simulink model "Template_v5_0_0_2024b_Jetson"  (R2024b)
settings: Solver=ode4  StartTime=0.0  StopTime=tsim  FixedStep=baseRate  RelTol=1e-6  AbsTol=1e-6
values from neighbouring files (symbols this model uses):
  Gamma1_el = 0.12    [Run_Initializer.m]
  Gamma1_sh = 0.005    [Run_Initializer.m]
  Gamma1_wr = 0.025    [Run_Initializer.m]
  Gamma2_el = 5    [Run_Initializer.m]
  Gamma2_sh = 5    [Run_Initializer.m]
  Gamma2_wr = 5    [Run_Initializer.m]
  Gamma3_el = 10    [Run_Initializer.m]
  Gamma3_sh = 40    [Run_Initializer.m]
  Gamma3_wr = 40    [Run_Initializer.m]
  Gamma4_el = 0.039    [Run_Initializer.m]
  Gamma4_sh = 0.015    [Run_Initializer.m]
  Gamma4_wr = 0.029    [Run_Initializer.m]
  Gamma5_el = 800    [Run_Initializer.m]
  Gamma5_sh = 800    [Run_Initializer.m]
  Gamma5_wr = 800    [Run_Initializer.m]
  Gamma6_el = 0.000001    (= 1e-06)    [Run_Initializer.m]
  Gamma6_sh = 0.005    [Run_Initializer.m]
  Gamma6_wr = 0.02    [Run_Initializer.m]
  Kd_elarm = 0.8    [Run_Initializer.m]
  Kd_sharm = 1.0    (= 1)    [Run_Initializer.m]
  Kd_wrarm = 0.6    [Run_Initializer.m]
  Kp_elarm = 1.2    [Run_Initializer.m]
  Kp_sharm = 1.5    [Run_Initializer.m]
  Kp_wrarm = 1.0    (= 1)    [Run_Initializer.m]
  PWMFreq = 5    [Run_Initializer.m]
  Tz_lim_elarm = .1    (= 0.1)    [Run_Initializer.m]
  Tz_lim_sharm = .1    (= 0.1)    [Run_Initializer.m]
  Tz_lim_wrarm = .1    (= 0.1)    [Run_Initializer.m]
undefined symbols (not defined in the file or in its folder): a1, a2, a3, b0, b1, b2, b3, baseRate, dataRate, DiscIntNeverNeededParam, drop_states_ARM, drop_states_BLACK, drop_states_BLUE, drop_states_RED, F_red_X_nominal, F_red_Y_nominal, F_thrusters_BLACK, F_thrusters_BLUE, F_thrusters_RED, home_states_BLACK, home_states_BLUE, home_states_RED, IBLACK, IBLUE, IDIST, IEE, init_states_BLACK, init_states_BLUE, init_states_RED, IPROX, IRED, K_BLACK, K_BLUE, K_RED, Kd_tb, Kd_tblue, Kd_tr, Kd_xb, Kd_xblue, Kd_xr, Kd_yb, Kd_yblue, Kd_yr, Kp_tb, Kp_tblue, Kp_tr, Kp_xb, Kp_xblue, Kp_xr, Kp_yb, Kp_yblue, Kp_yr, mBLACK, mBLUE, mDIST, mEE, mPROX, mRED, Phase0_End, Phase1_End ... (+17)
libraries: simulink x30, nvidiaSharedBlocks x19, MainLibrary x5, dspinverses x3
(part 8 of 8)

== matlab function Template_v5_0_0_2024b_Jetson/Thruster & Float Control Code/Change RED Behavior/Calculate Duty Cycle/MATLAB Function5 ==
  data: H_final output; u_desired input; duty_cycles output; x0 input; thruster_dist2CG_RED parameter; F_red_X_nominal parameter; F_red_Y_nominal parameter; max_iters parameter; tol parameter
function [H_final, duty_cycles] = optimize_duty_cycle_with_decay( ...
    u_desired, x0, thruster_dist2CG_RED, F_red_X_nominal, F_red_Y_nominal, max_iters, tol)
    %OPTIMIZE_DUTY_CYCLE_WITH_DECAY 
    %   Iteratively optimizes thruster duty cycles while updating thrust decay.
    %
    %   Inputs:
    %       u_desired           - Desired force/torque vector [Fx; Fy; M] (3x1)
    %       x0                  - Initial guess for duty cycles (8x1)
    %       thruster_dist2CG_RED- Distances of thrusters from CG (vector, mm)
    %       F_red_X_nominal     - Nominal X-direction thruster force (scalar, N)
    %       F_red_Y_nominal     - Nominal Y-direction thruster force (scalar, N)
    %       max_iters           - Maximum optimization iterations
    %       tol                 - Convergence tolerance (on duty cycles)
    %
    %   Outputs:
    %       H_final     - Final H-matrix including thrust decay (3x8)
    %       duty_cycles - Optimized duty cycles (8x1)
    %

    % ---------------------------
    % Initialization
    % ---------------------------
    num_thrusters      = length(x0); %#ok<NASGU> % reserved if needed later
    duty_cycles        = x0;                     % current solution
    thrust_decay_factor = 1;                     % initial decay
    prev_duty_cycles   = duty_cycles + 2*tol;    % force first iteration

    % ---------------------------
    % Iterative optimization
    % ---------------------------
    for iter = 1:max_iters
        % Build system matrix H with current decay factor
        H = MakeHWithDecay(thruster_dist2CG_RED, F_red_X_nominal, ...
                           thrust_decay_factor, F_red_Y_nominal);

        % Solve constrained least squares (box constraints: 0 ≤ x ≤ 1)
        duty_cycles = custom_constrained_least_squares(H, u_desired, duty_cycles);

        % Update decay factor based on the current duty cycles
        [thrust_decay_factor, ~] = check_thrust_decay(duty_cycles);

        % Check convergence (∞-norm difference)
        if norm(duty_cycles - prev_duty_cycles, Inf) < tol
            H_final = MakeHWithDecayRecalculateForce(thruster_dist2CG_RED, ...
                        F_red_X_nominal, thrust_decay_factor, F_red_Y_nominal);
            return;
        end

        % Update reference for next iteration
        prev_duty_cycles = duty_cycles;
    end

    % If not converged within max_iters, return final H with last decay
    H_final = MakeHWithDecayRecalculateForce(thruster_dist2CG_RED, ...
                F_red_X_nominal, thrust_decay_factor, F_red_Y_nominal);
end


% ========================================================================
% Custom Constrained Least Squares Solver
% ========================================================================
function x_opt = custom_constrained_least_squares(H, b, x0)
    %CUSTOM_CONSTRAINED_LEAST_SQUARES
    %   Solves min_x ||H*x - b||^2 subject to 0 <= x <= 1
    %   using projected gradient descent with backtracking line search.
    %
    %   Inputs:
    %       H   - System matrix (3x8)
    %       b   - Desired vector (3x1)
    %       x0  - Initial guess (8x1)
    %
    %   Output:
    %       x_opt - Optimal duty cycle vector (8x1)

    % Parameters
    max_iterations = 100;
    tolerance      = 1e-6;
    alpha          = 0.01;  % initial step size
    beta           = 0.5;   % backtracking factor

    % Initialization
    x      = x0;
    x_prev = x0 + 2*tolerance;

    % Precompute matrices
    HtH = H' * H;
    Htb = H' * b;

    for iter = 1:max_iterations
        % Gradient of ||H*x - b||^2
        gradient = 2 * (HtH*x - Htb);

        % Store objective for comparison
        current_obj = norm(H*x - b)^2;

        % Backtracking line search
        step_size = alpha;
        for ls_iter = 1:20
            x_new = x - step_size * gradient;
            x_new = max(0, min(1, x_new)); % project into [0,1]

            new_obj = norm(H*x_new - b)^2;
            if new_obj < current_obj
                break; % accept step
            else
                step_size = step_size * beta;
            end
        end

        % Update
        x = x_new;

        % Convergence check
        if norm(x - x_prev) < tolerance
            break;
        end

        % Adaptive step size tuning
        if iter > 1 && new_obj < current_obj
            alpha = min(alpha * 1.1, 0.1); % speed up if progress
        else
            alpha = alpha * 0.9;           % slow down otherwise
        end

        % Store for next iteration
        x_prev = x;
    end

    x_opt = x;
end


% ========================================================================
% Construct H-matrix (with decay factor)
% ========================================================================
function H = MakeHWithDecay(thruster_dist2CG, F_X_nominal, thrust_decay_factor, F_Y_nominal)
    %MAKEHWITHDECAY
    %   Builds the H matrix that maps thruster duty cycles to [Fx; Fy; M],
    %   applying thrust decay.
    %
    %   Outputs H as (3x8)

    % Convert thruster arm distances to meters
    adjusted_dist = thruster_dist2CG / 1000;

    % Thruster directions (X, Y, and moment arm)
    Vec1 = [-1; -1;  0;  0;  1;  1;  0;  0]; % X
    Vec2 = [ 0;  0;  1;  1;  0;  0; -1; -1]; % Y
    Vec3 = adjusted_dist;                    % moment (Z)

    Mat1 = [Vec1, Vec2, Vec3]';

    % Thruster forces (scaled by decay)
    F_thrusters = [F_X_nominal; F_X_nominal; ...
                   F_Y_nominal; F_Y_nominal; ...
                   F_X_nominal; F_X_nominal; ...
                   F_Y_nominal; F_Y_nominal] * thrust_decay_factor;

    % Build diagonal scaling
    Mat2 = diag(F_thrusters / 2);

    % Final mapping
    H = Mat1 * Mat2;
end


% ========================================================================
% Construct H-matrix (recalculate full force with decay)
% ========================================================================
function H = MakeHWithDecayRecalculateForce(thruster_dist2CG, F_X_nominal, thrust_decay_factor, F_Y_nominal)
    %MAKEHWITHDECAYRECALCULATEFORCE
    %   Same as MakeHWithDecay but applies full nominal force scaling.

    adjusted_dist = thruster_dist2CG / 1000;

    Vec1 = [-1; -1;  0;  0;  1;  1;  0;  0];
    Vec2 = [ 0;  0;  1;  1;  0;  0; -1; -1];
    Vec3 = adjusted_dist;

    Mat1 = [Vec1, Vec2, Vec3]';

    F_thrusters = [F_X_nominal; F_X_nominal; ...
                   F_Y_nominal; F_Y_nominal; ...
                   F_X_nominal; F_X_nominal; ...
                   F_Y_nominal; F_Y_nominal] * thrust_decay_factor;

    Mat2 = diag(F_thrusters);

    H = Mat1 * Mat2;
end


% ========================================================================
% Thrust Decay Update Rule
% ========================================================================
function [thrust_decay_factor, count] = check_thrust_decay(PWMs)
    %CHECK_THRUST_DECAY
    %   Updates thrust decay factor based on average duty cycle.
    %
    %   Inputs:
    %       PWMs - Duty cycle vector (8x1)
    %
    %   Outputs:
    %       thrust_decay_factor - Adjusted decay factor (scalar)
    %       count               - Number of active thrusters

    % Normalize if needed
    if max(PWMs) > 1
        PWMs = PWMs / max(PWMs);
    end
    
    % Active thrusters
    count = sum(PWMs > 0);
    
    % Mean duty cycle (only active thrusters)
    avg_duty = sum(max(PWMs, 0)) / max(count, 1);
    
    % Update rule (piecewise)
    if avg_duty < 0.3 || count == 0
        thrust_decay_factor = 1;
    else
        thrust_decay_factor = max(0.6 - 2*avg_duty + 1, 0.5);
    end
end

== matlab function Template_v5_0_0_2024b_Jetson/Thruster & Float Control Code/Change RED Behavior/Calculate Duty Cycle/Rotate Forces to Inertial/Create Rotation Matrix ==
  data: Rz input; C_Ib output
function C_Ib = RotateFrame(Rz)

C_bI = [  cos(Rz) sin(Rz)
         -sin(Rz) cos(Rz) ];

C_Ib = inv(C_bI);

end

== matlab function Template_v5_0_0_2024b_Jetson/Thruster & Float Control Code/Change RED Behavior/Rotate Forces to Body/Create Rotation Matrix ==
  data: Rz input; C_bI output
function C_bI = RotateFrame(Rz)

C_bI = [  cos(Rz) sin(Rz)
         -sin(Rz) cos(Rz) ];

end

== matlab function Template_v5_0_0_2024b_Jetson/Thruster & Float Control Code/Change BLACK Behavior/Calculate Duty Cycle/MATLAB Function1 ==
  data: ThrustPer_Final output; ThrustPer input; PWMFreq parameter
function ThrustPer_Final  = ThrusterSat(ThrustPer, PWMFreq)

    ValveTime       = 0.007;
    TControl        = 1/PWMFreq;

    ThrustPer_Final = zeros(8,1);
    
    if max(ThrustPer) > 1
        ThrustPer_Sat = ThrustPer/max(ThrustPer);
    else
        ThrustPer_Sat = ThrustPer;
    end
    
    for i = 1:8
        if ThrustPer_Sat(i) > ValveTime/TControl 
            ThrustPer_Final(i) = ThrustPer_Sat(i);
        else
            ThrustPer_Final(i) = 0;
        end
    end


end

== matlab function Template_v5_0_0_2024b_Jetson/Thruster & Float Control Code/Change RED Behavior/Calculate Duty Cycle/MATLAB Function8 ==
  data: ThrustPer_Final output; ThrustPer input; PWMFreq parameter
function ThrustPer_Final  = ThrusterSat(ThrustPer, PWMFreq)

    ValveTime       = 0.007;
    TControl        = 1/PWMFreq;

    ThrustPer_Final = zeros(8,1);
    
    if max(ThrustPer) > 1
        ThrustPer_Sat = ThrustPer/max(ThrustPer);
    else
        ThrustPer_Sat = ThrustPer;
    end
    
    for i = 1:8
        if ThrustPer_Sat(i) > ValveTime/TControl 
            ThrustPer_Final(i) = ThrustPer_Sat(i);
        else
            ThrustPer_Final(i) = 0;
        end
    end


end

== matlab function Template_v5_0_0_2024b_Jetson/Simulate Plant Dynamics/RED and ARM Dynamics/RED + ARM/Dynamics Model ==
  data: q_dot output; x input; InertiaS input; CoriolisS input; u input; Gamma1_sh parameter; Gamma2_sh parameter; Gamma3_sh parameter; Gamma5_sh parameter; Gamma4_sh parameter; Gamma6_sh parameter; Gamma1_el parameter; Gamma2_el parameter; Gamma3_el parameter; Gamma5_el parameter; Gamma4_el parameter; Gamma6_el parameter; Gamma1_wr parameter; Gamma2_wr parameter; Gamma3_wr parameter; Gamma5_wr parameter; Gamma4_wr parameter; Gamma6_wr parameter; q_ddot output
function [q_dot, q_ddot]  = DynamicsModel(x, InertiaS, CoriolisS, u,...
    Gamma1_sh, Gamma2_sh, Gamma3_sh, Gamma5_sh, Gamma4_sh, Gamma6_sh,...
    Gamma1_el, Gamma2_el, Gamma3_el, Gamma5_el, Gamma4_el, Gamma6_el,...
    Gamma1_wr, Gamma2_wr, Gamma3_wr, Gamma5_wr, Gamma4_wr, Gamma6_wr)


    fqdot1 = Gamma1_sh*(tanh(Gamma2_sh*x(10)) - tanh(Gamma3_sh*x(10))) + Gamma4_sh*tanh(Gamma5_sh*x(10)) + Gamma6_sh*x(10);

    fqdot2 = Gamma1_el*(tanh(Gamma2_el*x(11)) - tanh(Gamma3_el*x(11))) + Gamma4_el*tanh(Gamma5_el*x(11)) + Gamma6_el*x(11);

    fqdot3 = Gamma1_wr*(tanh(Gamma2_wr*x(12)) - tanh(Gamma3_wr*x(12))) + Gamma4_wr*tanh(Gamma5_wr*x(12)) + Gamma6_wr*x(12);
    
    q_dot  = x(7:12);
    q_ddot = pinv(InertiaS)*(u - CoriolisS*x(7:12) - [0;0;0;fqdot1;fqdot2;fqdot3]);
    
end

== matlab function Template_v5_0_0_2024b_Jetson/Simulate Plant Dynamics/RED and ARM Dynamics/RED Only/Calculated & Store Measured States/Subsystem1/Enabled Subsystem/MATLAB Function ==
  data: y input; dy output; dt input; tau input; ema_prev input; ema output
function [dy, ema] = realtime_derivative_ema(y, dt, tau, ema_prev)
    % Compute smoothed derivative using Exponential Moving Average
    %
    % Inputs:
    %   y        : Current measurement
    %   dt       : Time step
    %   tau      : Time constant for EMA filter (larger = more smoothing)
    %   ema_prev : Previous EMA value
    %
    % Outputs:
    %   dy  : Smoothed derivative estimate
    %   ema : Updated EMA value
    
    % Calculate smoothing factor from time constant
    alpha = 1 - exp(-dt ./ tau);
    
    % Update Exponential Moving Average
    ema = alpha .* y + (1 - alpha) .* ema_prev;
    
    % Compute derivative using finite difference on smoothed values
    dy = (ema - ema_prev) ./ dt;
end

== matlab function Template_v5_0_0_2024b_Jetson/Thruster & Float Control Code/Change BLUE Behavior/Calculate Duty Cycle/MATLAB Function1 ==
  data: ThrustPer_Final output; ThrustPer input; PWMFreq parameter
function ThrustPer_Final  = ThrusterSat(ThrustPer, PWMFreq)

    ValveTime       = 0.007;
    TControl        = 1/PWMFreq;

    ThrustPer_Final = zeros(8,1);
    
    if max(ThrustPer) > 1
        ThrustPer_Sat = ThrustPer/max(ThrustPer);
    else
        ThrustPer_Sat = ThrustPer;
    end
    
    for i = 1:8
        if ThrustPer_Sat(i) > ValveTime/TControl 
            ThrustPer_Final(i) = ThrustPer_Sat(i);
        else
            ThrustPer_Final(i) = 0;
        end
    end


end

== matlab function Template_v5_0_0_2024b_Jetson/3 - Control/Default LQR Control (RED)/Calculate Error/MATLAB Function ==
  data: Rz_path input; Rz_error output; Rz_measured input
function Rz_error = SmoothAngularDifference(Rz_path, Rz_measured)

    Rz_error = mod(Rz_measured-Rz_path+pi, 2*pi)-pi;


end

== matlab function Template_v5_0_0_2024b_Jetson/3 - Control/Default LQR Control (BLACK)/Calculate Error/MATLAB Function ==
  data: Rz_path input; Rz_error output; Rz_measured input
function Rz_error = SmoothAngularDifference(Rz_path, Rz_measured)

    Rz_error = mod(Rz_measured-Rz_path+pi, 2*pi)-pi;


end

== matlab function Template_v5_0_0_2024b_Jetson/3 - Control/Default PD Control (RED)/Calculate Error/MATLAB Function ==
  data: Rz_path input; Rz_error output; Rz_measured input
function Rz_error = SmoothAngularDifference(Rz_path, Rz_measured)

    Rz_error = mod(Rz_measured-Rz_path+pi, 2*pi)-pi;


end

== matlab function Template_v5_0_0_2024b_Jetson/3 - Control/Default PD Control (BLACK)/Calculate Error/MATLAB Function ==
  data: Rz_path input; Rz_error output; Rz_measured input
function Rz_error = SmoothAngularDifference(Rz_path, Rz_measured)

    Rz_error = mod(Rz_measured-Rz_path+pi, 2*pi)-pi;


end
